simulink model "MPPT using Simulink"  (R2016a)
settings: Solver=VariableStepAuto  StartTime=0.0  StopTime=0.5  RelTol=1e-3
libraries: powerlib x9, simulink x2, re_lib x1
settings Model: Creator=win10  LastModifiedBy=win10

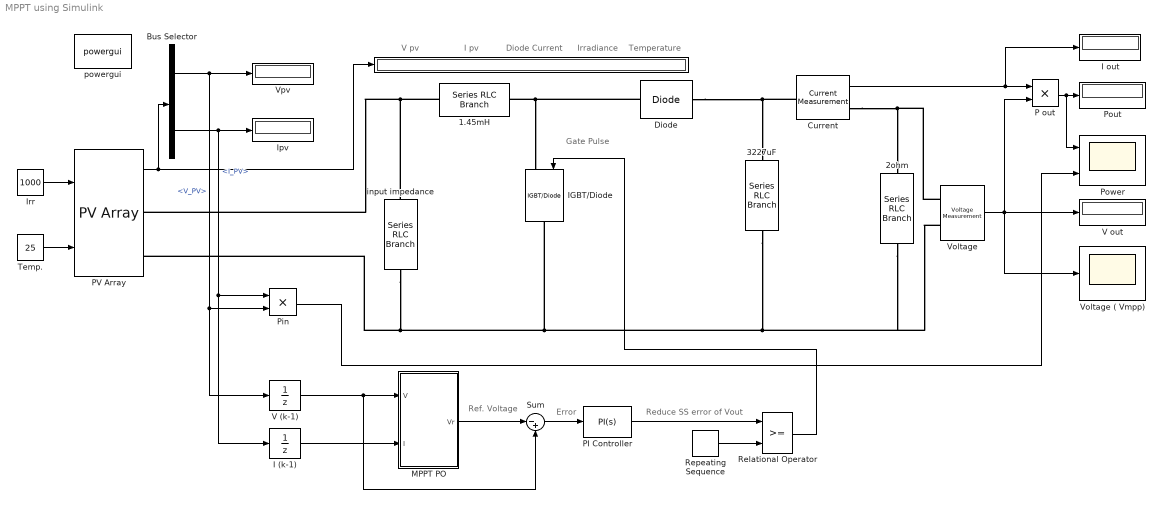
== system MPPT using Simulink ==
  note: Temperature
  note: Irradiance
  note: Diode Current
  note: I pv
  note: V pv
  note: Reduce SS error of Vout
  note: Ref. Voltage
  note: Gate Pulse
  note: Error
  "                                                                                            " : Display
      settings: Decimation=2
  1.45mH : powerlib/Elements/Series RLC Branch  LConnTagsString=__new0  RConnTagsString=__new0  BranchType=L  Resistance=1  Inductance=1.45e-3  SetiL0=off  InitialCurrent=0  Capacitance=1e-6  Setx0=off  InitialVoltage=0  Measurements=Branch current
  2ohm : powerlib/Elements/Series RLC Branch  LConnTagsString=__new0  RConnTagsString=__new0  BranchType=R  Resistance=2  Inductance=1e-3  SetiL0=off  InitialCurrent=0  Capacitance=1e-6  Setx0=off  InitialVoltage=0  Measurements=Branch voltage
  3227uF : powerlib/Elements/Series RLC Branch  LConnTagsString=__new0  RConnTagsString=__new0  BranchType=C  Resistance=1  Inductance=1e-3  SetiL0=off  InitialCurrent=0  Capacitance=3227e-6  Setx0=off  InitialVoltage=0  Measurements=Branch voltage
  Bus Selector : BusSelector  OutputSignals=V_PV,I_PV
  "Current " : powerlib/Measurements/Current Measurement  PhasorSimulation=off  OutputType=Complex  PSBequivalent=0
  Diode : powerlib/Power Electronics/Diode  Ron=0.001  Lon=0  Vf=0.7  IC=0  UseSnubber=off  Rs=500  Cs=250e-9  Measurements=off
  I (k-1) : UnitDelay  SampleTime=1e-4
  I out : Display
      settings: Decimation=2
  IGBT/Diode : powerlib/Power Electronics/IGBT//Diode  Ron=1e-3  Rs=1e5  Cs=inf  Measurements=off
  Ipv : Display
      settings: Decimation=2
  Irr : Constant  Value=1000
  MPPT PO : MATLAB Function  TreatAsAtomicUnit=on
  P out : Product
  PI Controller : simulink/Continuous/PID Controller  Controller=PI  TimeDomain=Continuous-time  SampleTime=-1  IntegratorMethod=Forward Euler  FilterMethod=Forward Euler  Form=Ideal  UseFilter=on  ControllerParametersSource=internal  P=0.001  I=0.01  D=0  N=100  InitialConditionSource=internal  InitialConditionForIntegrator=0  InitialConditionForFilter=0  ExternalReset=none  LimitOutput=on  UpperSaturationLimit=0.95  LowerSaturationLimit=0  LinearizeAsGain=on  AntiWindupMode=none  Kb=1  TrackingMode=off  Kt=1  PParamMin=[]  PParamMax=[]  IParamMin=[]  IParamMax=[]  DParamMin=[]  DParamMax=[]  NParamMin=[]  NParamMax=[]  KbParamMin=[]  KbParamMax=[]  KtParamMin=[]  KtParamMax=[]  POutMin=[]  POutMax=[]  IOutMin=[]  IOutMax=[]  DOutMin=[]  DOutMax=[]  NOutMin=[]  NOutMax=[]  KbOutMin=[]  KbOutMax=[]  KtOutMin=[]  KtOutMax=[]  IntegratorOutMin=[]  IntegratorOutMax=[]  FilterOutMin=[]  FilterOutMax=[]  SumOutMin=[]  SumOutMax=[]  SumI1OutMin=[]  SumI1OutMax=[]  SumI2OutMin=[]  SumI2OutMax=[]  SumI3OutMin=[]  SumI3OutMax=[]  SumDOutMin=[]  SumDOutMax=[]  SaturationOutMin=[]  SaturationOutMax=[]  IntegratorContinuousStateAttributes=''  IntegratorStateMustResolveToSignalObject=off  IntegratorRTWStateStorageClass=Auto  FilterContinuousStateAttributes=''  FilterStateMustResolveToSignalObject=off  FilterRTWStateStorageClass=Auto  DifferentiatorICPrevScaledInput=0  DifferentiatorOutMin=[]  DifferentiatorOutMax=[]
  PV Array : re_lib/Solar/PV Array  Npar=50  Nser=10  PlotType=array @ 25 deg.C & specified irradiances  S_vec="[ 3000  800 600 400 300 ]"  Temp_C_vec="[ 45 40 38 32 25  ]"  ModuleName=1Soltech 1STH-215-P  PlotWhenSelected=off  Pm=213.15  Ncell=60  Voc=36.3  Isc=7.84  Vm=29  Im=7.35  beta_Voc_pc=-0.36099  alpha_Isc_pc=0.102  beta_Voc=-0.13104  alpha_Isc=0.007997  IL=7.8649  I0=2.9259e-10  nI=0.98117  Rsh=313.3991  Rs=0.39383  BAL=off  Tc=1e-6  Tfilter=5e-5
  Pin : Product
  Pout : Display
      settings: Decimation=2
  Power : Scope  NumInputPorts=2
  Relational Operator : RelationalOperator  OutDataTypeStr=boolean
  Repeating Sequence : simulink/Sources/Repeating Sequence  rep_seq_t=[0 0.2]/1000  rep_seq_y="[ 0 1  ]"
  Sum : Sum  Inputs=|-+
  Temp. : Constant  Value=25
  V (k-1) : UnitDelay  SampleTime=1e-4
  V out : Display
      settings: Decimation=2
  "Voltage " : powerlib/Measurements/Voltage Measurement  PhasorSimulation=off  OutputType=Complex  PSBequivalent=0
  Voltage ( Vmpp) : Scope
  Vpv : Display
      settings: Decimation=2
  input impedance : powerlib/Elements/Series RLC Branch  LConnTagsString=__new0  RConnTagsString=__new0  BranchType=RC  Resistance=0.0001  Inductance=1e-3  SetiL0=off  InitialCurrent=0  Capacitance=1000e-6  Setx0=off  InitialVoltage=0  Measurements=Branch voltage
  powergui : powerlib/powergui  Priority=1  SimulationMode=Discrete  SolverType=Tustin/Backward Euler (TBE)  SampleTime=1e-6  frequency=60  SPID=off  DisableSnubberDevices=on  DisableRonSwitches=on  DisableVfSwitches=on  SwTol=0  DisplayEquations=off  Interpol=off  ExternalGateDelay=off  methode=off  Ts=10  FunctionMessages=off  echomessages=off  HookPort=off  EnableUseOfTLC=off  x0status=blocks  frequencyindice=0  Pbase=100e6  ErrMax=1e-4  Iterations=50  UnitsV=kV  UnitsW=MW  buscounter=0  RestoreLinks=warning  ResistiveCurrentMeasurement=off  Frange=[0:2:500]  Ylog=off  Xlog=on  ShowGrid=off  save=off  variable=ZData  structure=0  ZoomFFT=off  StartTime=0.0  cycles=1  DisplayStyle=1  fundamental=60  FreqAxis=off  MaxFrequency=1000  frequencyindicesteady=1  RmsSteady=1  display=off
  wires:
  Irr/1 -> PV Array/1
  Temp./1 -> PV Array/2
  PV Array/1 -> "                                                                                            "/1, Bus Selector/1
  Bus Selector/2 -> Pin/1, I (k-1)/1, Ipv/1  "<I_PV>"
  Bus Selector/1 -> Pin/2, V (k-1)/1, Vpv/1  "<V_PV>"
  MPPT PO/1(Vr) -> Sum/1
  Sum/1 -> PI Controller/1
  P out/1 -> Power/1, Pout/1
  PI Controller/1 -> Relational Operator/1
  Repeating Sequence/1 -> Relational Operator/2
  "Current "/1 -> I out/1, P out/1
  "Voltage "/1 -> P out/2, Voltage ( Vmpp)/1, V out/1
  Relational Operator/1 -> IGBT/Diode/1
  V (k-1)/1 -> Sum/2, MPPT PO/1(V)
  I (k-1)/1 -> MPPT PO/2(I)
  Pin/1 -> Power/2
  connections:
  Diode/LConn1 -- IGBT/Diode/LConn1 -- 1.45mH/RConn1
  2ohm/RConn1 -- "Voltage "/LConn2 -- 3227uF/RConn1 -- IGBT/Diode/RConn1 -- input impedance/RConn1 -- PV Array/RConn2
  Diode/RConn1 -- 3227uF/LConn1 -- "Current "/LConn1
  "Current "/RConn1 -- 2ohm/LConn1 -- "Voltage "/LConn1
  1.45mH/LConn1 -- input impedance/LConn1 -- PV Array/RConn1

== matlab function MPPT using Simulink/MPPT PO ==
  data: V input; I input; Vr output
function Vr = MPPTPO(V, I)

Vrmax=363;     % from PV array configuration
Vrmin=0;
Vrini=250;     % initial value of Vref , nearer to Vmpp
del_Vr=3;      % perturb value of Vref
persistent Vold Pold Vrold;

if isempty(Vold)       % Run only at once 
    Vold=0;
    Pold=0;
    Vrold = Vrini;
end

P=V*I;
dV=V-Vold;

if (P ~= Pold)
   if (P<Pold) 
        if (V<Vold)
             Vr=Vrold+del_Vr;
        else Vr=Vrold-del_Vr;
        end
    
   else 
        if (V<Vold)
             Vr=Vrold-del_Vr;
        else Vr=Vrold+del_Vr;
        end
   end
else Vr=Vrold;
end

if Vr >= Vrmax | Vr<=Vrmin 
    Vr= Vrold;
end

Vrold =Vr;
Vold=V;
Pold=P;
